simulink model "L5T1_SinglePhaseHBridge"  (R2021a)
settings: Solver=VariableStepAuto  StartTime=0.0  StopTime=0.06  RelTol=1e-3  EnableMultiTasking=on
libraries: spsIGBTDiodeLib x4, spsTriangleGeneratorLib x2, spsVoltageMeasurementLib x2, spsACVoltageSourceLib x1, spsCurrentMeasurementLib x1, spsDCVoltageSourceLib x1, spsSeriesRLCBranchLib x1, spspowerguiLib x1
settings Model: Creator=User  LastModifiedBy=hp
settings SolverCC: AlgebraicLoopSolver=TrustRegion
settings DataIOCC: ReturnWorkspaceOutputs=off
settings OptimizationCC: LifeSpan=inf
settings DebuggingCC: SFUnexpectedBacktrackingDiag=warning  SFNoUnconditionalDefaultTransitionDiag=warning  SFMachineParentedDataDiag=warning  ArithmeticOperatorsInVariantConditions=warning
settings SFSimCC: SimUseLocalCustomCode=off  CustomCodeUndefinedFunction=UseInterfaceOnly
settings RTWCC: RTWUseLocalCustomCode=off
settings CodeAppCC: StateflowObjectComments=on
settings GRTTargetCC: TargetLangStandard=C89/C90 (ANSI)
settings ConfigComp: CovMetricSettings=dw  CovSaveCumulativeToWorkspaceVar=on  CovSaveSingleToWorkspaceVar=on  CovExternalEMLEnable=off
settings SimscapeCC: SimscapeNormalizeSystem=off

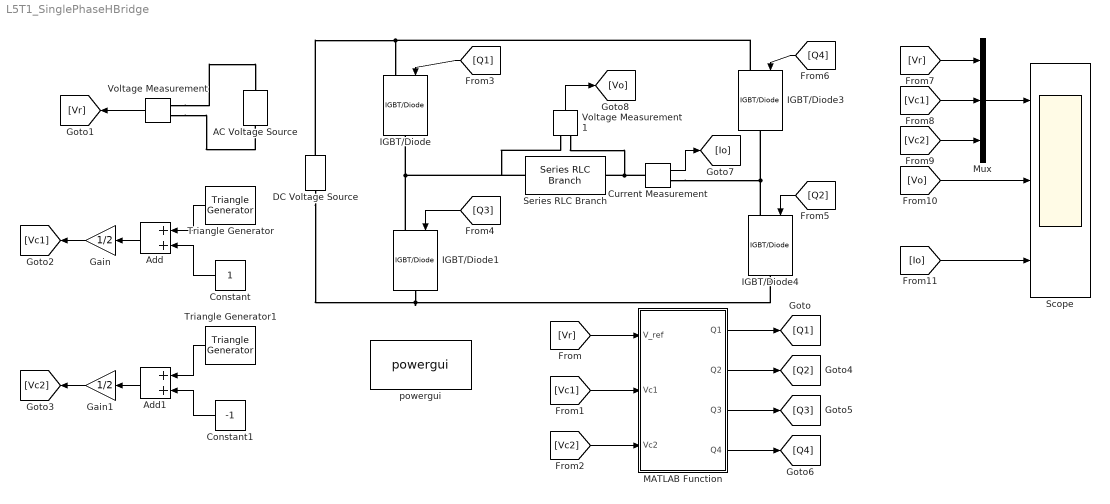
== system L5T1_SinglePhaseHBridge ==
  AC Voltage Source : spsACVoltageSourceLib/AC Voltage Source  Amplitude=1  Phase=0  Frequency=50  SampleTime=0  Measurements=None  BusType=swing  Pref=10e3  Qref=0  Qmin=-inf  Qmax=+inf
  Add : Sum
  Add1 : Sum
  Constant : Constant
  Constant1 : Constant  Value=-1
  Current Measurement : spsCurrentMeasurementLib/Current Measurement  PhasorSimulation=off  OutputType=Complex  PSBequivalent=0
  DC Voltage Source : spsDCVoltageSourceLib/DC Voltage Source  Amplitude=100  Measurements=None
  Gain : Gain  Gain=1/2
  Gain1 : Gain  Gain=1/2
  IGBT/Diode{,1,3..4} (4 alike) : spsIGBTDiodeLib/IGBT//Diode  Ron=1e-3  Rs=1e5  Cs=inf  Measurements=off
  MATLAB Function : MATLAB Function  TreatAsAtomicUnit=on
  Mux : Mux  Inputs=3
  Scope : Scope  NumInputPorts=3
  Series RLC Branch : spsSeriesRLCBranchLib/Series RLC Branch  LConnTagsString=__new0  RConnTagsString=__new0  BranchType=RL  Resistance=10  Inductance=100e-3  SetiL0=off  InitialCurrent=0  Capacitance=1e-6  Setx0=off  InitialVoltage=0  Measurements=None
  Triangle Generator : spsTriangleGeneratorLib/Triangle Generator  Freq=1500  Phase=0  Ts=0
  Triangle Generator1 : spsTriangleGeneratorLib/Triangle Generator  Freq=1500  Phase=180  Ts=0
  Voltage Measurement : spsVoltageMeasurementLib/Voltage Measurement  PhasorSimulation=off  OutputType=Complex  PSBequivalent=0
  Voltage Measurement1 : spsVoltageMeasurementLib/Voltage Measurement  PhasorSimulation=off  OutputType=Complex  PSBequivalent=0
  powergui : spspowerguiLib/powergui  Priority=1  SimulationMode=Discrete  SampleTime=50e-6  frequency=60  Iterations=50  frequencyindice=0  Pbase=100e6  ErrMax=1e-4  UnitsV=kV  UnitsW=MW  buscounter=0  FunctionMessages=off  echomessages=off  EnableUseOfTLC=off  CurrentSourceSwitches=off  DisableSnubberDevices=off  DisableRonSwitches=off  DisableVfSwitches=off  DisplayEquations=off  AutomaticDiscreteSolvers=off  SolverType=Tustin/Backward Euler (TBE)  Interpol=off  ExternalGateDelay=off  methode=off  Ts=10  x0status=blocks  SPID=off  SwTol=0  HookPort=off  NonlinearTolerance=1e-4  nMaxIteration=100  ContinueOnMaxIteration=off  RestoreLinks=warning  ResistiveCurrentMeasurement=off  Frange=[0:2:500]  Ylog=off  Xlog=on  ShowGrid=off  save=off  variable=ZData  structure=0  ZoomFFT=off  StartTime=0.0  cycles=1  DisplayStyle=1  fundamental=60  FreqAxis=off  MaxFrequency=1000  frequencyindicesteady=1  RmsSteady=1  display=off
  wires:
  Triangle Generator/1 -> Add/1
  Constant/1 -> Add/2
  Triangle Generator1/1 -> Add1/1
  Constant1/1 -> Add1/2
  Add/1 -> Gain/1
  Add1/1 -> Gain1/1
  Mux/1 -> Scope/1
  Voltage Measurement/1 -> [Vr]
  Gain/1 -> [Vc1]
  Gain1/1 -> [Vc2]
  [Vr] -> MATLAB Function/1(V_ref)
  [Vc2] -> MATLAB Function/3(Vc2)
  [Vc1] -> MATLAB Function/2(Vc1)
  MATLAB Function/1(Q1) -> [Q1]
  MATLAB Function/2(Q2) -> [Q2]
  MATLAB Function/3(Q3) -> [Q3]
  MATLAB Function/4(Q4) -> [Q4]
  Voltage Measurement1/1 -> [Vo]
  Current Measurement/1 -> [Io]
  [Q1] -> IGBT/Diode/1
  [Q4] -> IGBT/Diode3/1
  [Q2] -> IGBT/Diode4/1
  [Q3] -> IGBT/Diode1/1
  [Vr] -> Mux/1
  [Vc1] -> Mux/2
  [Vc2] -> Mux/3
  [Vo] -> Scope/2
  [Io] -> Scope/3
  connections:
  Voltage Measurement/LConn1 -- AC Voltage Source/RConn1
  Voltage Measurement/LConn2 -- AC Voltage Source/LConn1
  IGBT/Diode1/LConn1 -- Series RLC Branch/LConn1 -- Voltage Measurement1/LConn1 -- IGBT/Diode/RConn1
  IGBT/Diode4/LConn1 -- Current Measurement/RConn1 -- IGBT/Diode3/RConn1
  DC Voltage Source/LConn1 -- IGBT/Diode1/RConn1 -- IGBT/Diode4/RConn1
  IGBT/Diode3/LConn1 -- DC Voltage Source/RConn1 -- IGBT/Diode/LConn1
  Current Measurement/LConn1 -- Voltage Measurement1/LConn2 -- Series RLC Branch/RConn1

== matlab function L5T1_SinglePhaseHBridge/MATLAB Function ==
  data: V_ref input; Q1 output; Q2 output; Q3 output; Q4 output; Vc1 input; Vc2 input
function [Q1,Q2,Q3,Q4] = fcn(V_ref,Vc1,Vc2)
if V_ref>=0
    if V_ref>=Vc1
    Q1=1;
    Q2=1;
    Q3=0;
    Q4=0;
    else
    Q1=1;
    Q2=0;
    Q3=0;
    Q4=1;
    end
else
    if V_ref<=Vc2
    Q1=0;
    Q2=0;
    Q3=1;
    Q4=1;
    else
    Q1=0;
    Q2=1;
    Q3=1;
    Q4=0;
    end
end
end
